simulink model "AIV_robot"  (R2024b)
settings: Solver=VariableStepAuto  StartTime=0.0  StopTime=35  RelTol=1e-2
InitFcn:
  | %% Position Error parameter
  | goal_x = 18.5;
  | goal_y = 16;
  | 
  | s0 = sqrt(goal_x^2 + goal_y^2);
  | isGoal_dist = 1.0;
  | 
  | %% Velocity parameter
  | VelScaler = 15;
  | 
  | 
  | %% get bus
  | BusActors = Simulink.Bus;
  | BusActors = getBusActors(BusActors);
  | BusActorsActors = Simulink.Bus;
  | BusActorsActors= getBusActorsActors(BusActorsActors);
  | 
  | %% get agent
  | load("agent.mat")
model workspace (MAT data in the model file):
  firstWarning = 1
  originalScenarioChecksum = '7C1E912B2141DACB6907C14F620C989B'
libraries: simulink x13, drivingscenarioandsensors x8, simulink_extras x1, autolibshared x1, rllib x1
(part 9 of 9)

== matlab function AIV_robot/Environment/Simulation/Radar Sensor Processing/radar_scaling ==
  data: u input; u output
function u = radar_processing(u)

for i = 1:10
    if u(i) == 0
        u(i) = 10;
    end
    u(i) = u(i) / 10;
end

== matlab function AIV_robot/Environment/Simulation/Ultrasonic Sensor Processing/ultrasonic_scaling ==
  data: u input; u output
function u = ultrasonic_processing(u)

for i = 1:6
    if u(i) == 0
        u(i) = 5;
    end
    u(i) = u(i) / 5;
end

== matlab function AIV_robot/Environment/Simulation/Ultrasonic Sensor Processing/prev_ultrasonic_scaling ==
  data: u input; u output
function u = ultrasonic_processing(u)

for i = 1:6
    if u(i) == 0
        u(i) = 5;
    end
    u(i) = u(i) / 5;
end

== matlab function AIV_robot/Environment/Simulation/Radar Sensor Processing/prev_radar_scaling ==
  data: u input; u output
function u = radar_processing(u)

for i = 1:10
    if u(i) == 0
        u(i) = 10;
    end
    u(i) = u(i) / 10;
end

== matlab function AIV_robot/Environment/Simulation/Pack Ego Actor ==
  data: pos input; egoActor output Bus: BusActorsActors size=1; vel input; yaw input; yawRate input; egoActorID input
function egoActor = packEgo(pos,vel,yaw,yawRate,egoActorID)

egoActor = struct(...
    'ActorID',egoActorID,...
    'Position', [pos(1) pos(2) 0], ...
    'Velocity', [vel(1) vel(2) 0], ...
    'Roll', 0, ...
    'Pitch', 0, ...
    'Yaw', yaw, ...
    'AngularVelocity', [0 0 yawRate]);
